simulink model "CA_CSE1_V1e_wo_LOSV2b"  (Simulink 7.3)
settings: Solver=ode3  StartTime=0.0  StopTime=Inf  FixedStep=0.1  RelTol=1e-3
undefined symbols (not defined in the file): eta1_0_real, v1_0_real, velocitySatValues1
libraries: simulink_extras x7, marine_gnc x5, simulink x5, dspinverses x2
(part 1 of 2)
settings Model: Creator=Dinh  LastModifiedBy=mcl  BufferReuse=off
settings DataIOCC: LimitDataPoints=off  SaveOutput=off  SaveTime=off
settings OptimizationCC: BlockReduction=off  BooleanDataType=off  ConditionallyExecuteInputs=off  OptimizeBlockIOStorage=off  BufferReuse=off  ExpressionFolding=off  LocalBlockOutputs=off  SimCompilerOptimization=On
settings SFSimCC: SimBuildMode=sf_nonincremental_build
settings RTWCC: SystemTargetFile=nidll.tlc  TemplateMakefile=nidll_vc.tmf  Description=NI Real-Time Target for Release 2007b or later  ProcessScript=nidll_make_rtw_hook
settings STFCustomTargetCC: MatFileLogging=on  SystemTargetFile=nidll.tlc

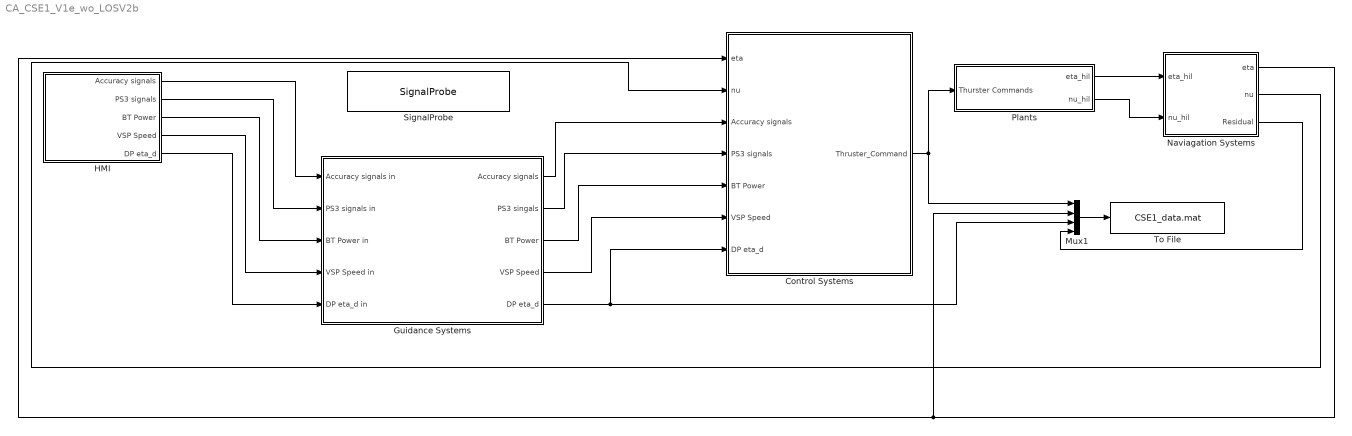
== system CA_CSE1_V1e_wo_LOSV2b ==
  Control Systems : Subsystem
  Guidance Systems : Subsystem
  HMI : Subsystem
  Mux1 : Mux
  Naviagation Systems : Subsystem
      settings: MinAlgLoopOccurrences=on
  Plants : Subsystem
  SignalProbe : S-Function  Description=Use this block with SIT.  FunctionName=SignalProbe  Parameters=1  EnableBusSupport=off
      settings: PreSaveFcn=NISIT_ModelVars;
      mask Description: The LabVIEW Simulation Interface Toolkit uses the SignalProbe block to probe the signals in the model. The SignalProbe block must be on the top level of the model hierarchy. You can have only one SignalProbe block per model file. Do not rename the SignalProbe block. Do not change the name of another model block to SignalProbe.
  To File : ToFile  Filename=CSE1_data.mat  MatrixName=cse1_data
  wires:
  Control Systems/1(Thruster_Command) -> Plants/1(Thurster Commands), Mux1/1
  HMI/2(PS3 signals) -> Guidance Systems/2(PS3 signals in)
  HMI/3(BT Power) -> Guidance Systems/3(BT Power in)
  HMI/4(VSP Speed) -> Guidance Systems/4(VSP Speed in)
  HMI/5(DP eta_d) -> Guidance Systems/5(DP eta_d in)
  Guidance Systems/2(PS3 singals) -> Control Systems/4(PS3 signals)
  Guidance Systems/3(BT Power) -> Control Systems/5(BT Power)
  Guidance Systems/4(VSP Speed) -> Control Systems/6(VSP Speed)
  Guidance Systems/5(DP eta_d) -> Control Systems/7(DP eta_d), Mux1/3
  Plants/1(eta_hil) -> Naviagation Systems/1(eta_hil)
  Plants/2(nu_hil) -> Naviagation Systems/2(nu_hil)
  Naviagation Systems/1(eta) -> Control Systems/1(eta), Mux1/2
  Naviagation Systems/2(nu) -> Control Systems/2(nu)
  Mux1/1 -> To File/1
  Guidance Systems/1(Accuracy signals) -> Control Systems/3(Accuracy signals)
  HMI/1(Accuracy signals) -> Guidance Systems/1(Accuracy signals in)
  Naviagation Systems/3(Residual) -> Mux1/4

== system CA_CSE1_V1e_wo_LOSV2b/Control Systems ==
  eta : Inport
  nu : Inport  Port=2
  Accuracy signals : Inport  Port=3
  PS3 signals : Inport  Port=4
  BT Power : Inport  Port=5
  VSP Speed : Inport  Port=6
  DP eta_d : Inport  Port=7
  Accuracy Control : Subsystem
  Control Switch : MultiPortSwitch  Inputs=4  zeroidx=on
  Control Mode : Constant  Value=0
  DP control : Subsystem
  Joystick Control : Subsystem
      settings: MinAlgLoopOccurrences=on
  Manual Thrust control : Subsystem
      settings: MinAlgLoopOccurrences=on
  Saturation : Saturate  UpperLimit=1.0  LowerLimit=-1.0
  if DP Control Mode : simulink/Logic and Bit Operations/Compare To Constant  SystemSampleTime=-1  relop===  const=3  LogicOutDataTypeMode=uint8
  Thruster_Command : Outport
  wires:
  PS3 signals/1 -> Manual Thrust control/1(PS3 Signals), Joystick Control/1(PS3 Signals)
  DP eta_d/1 -> DP control/1(eta_d)
  nu/1 -> DP control/3(nu)
  eta/1 -> DP control/2(eta)
  Control Mode/1 -> Control Switch/1, if DP Control Mode/1
  Control Switch/1 -> Saturation/1
  BT Power/1 -> Manual Thrust control/2(BT Power), Joystick Control/2(BT Power)
  VSP Speed/1 -> Manual Thrust control/3(VSP Speed), Joystick Control/3(VSP Speed)
  if DP Control Mode/1 -> DP control/Enable
  DP control/1(Thruster_Command_DP) -> Control Switch/5
  Joystick Control/1(Thruster_Command_Joystick) -> Control Switch/4
  Manual Thrust control/1(Thruster_Command_Manual) -> Control Switch/3
  Saturation/1 -> Thruster_Command/1
  Accuracy Control/1(Thruster Command Accuracy) -> Control Switch/2
  Accuracy signals/1 -> Accuracy Control/1(Accuracy signals)

== system CA_CSE1_V1e_wo_LOSV2b/Guidance Systems ==
  Accuracy signals in : Inport
  PS3 signals in : Inport  Port=2
  BT Power in : Inport  Port=3
  VSP Speed in : Inport  Port=4
  DP eta_d in : Inport  Port=5
  DP : Subsystem
  Demux1 : Demux  Outputs=3
  Mux : Mux  Inputs=3
  Terminator : Terminator
  psi_d : Gain  ParameterDataType=fixdt(1, 16)  ParameterScaling=2^0  OutDataType=fixdt(1, 16)  OutScaling=2^0
  x_d : Gain  ParameterDataType=fixdt(1, 16)  ParameterScaling=2^0  OutDataType=fixdt(1, 16)  OutScaling=2^0
  y_d : Gain  ParameterDataType=fixdt(1, 16)  ParameterScaling=2^0  OutDataType=fixdt(1, 16)  OutScaling=2^0
  Accuracy signals : Outport
  PS3 singals : Outport  Port=2
  BT Power : Outport  Port=3
  VSP Speed : Outport  Port=4
  DP eta_d : Outport  Port=5
  wires:
  DP eta_d in/1 -> DP/1(DP eta_d in)
  PS3 signals in/1 -> PS3 singals/1
  VSP Speed in/1 -> VSP Speed/1
  BT Power in/1 -> BT Power/1
  DP/1(DP eta_d) -> DP eta_d/1, Demux1/1
  Accuracy signals in/1 -> Accuracy signals/1
  x_d/1 -> Mux/1
  y_d/1 -> Mux/2
  psi_d/1 -> Mux/3
  Demux1/1 -> x_d/1
  Demux1/2 -> y_d/1
  Demux1/3 -> psi_d/1
  Mux/1 -> Terminator/1

== system CA_CSE1_V1e_wo_LOSV2b/HMI ==
  Accuracy control : Subsystem
  Battery Bow Thruster : Gain  ParameterDataType=fixdt(1, 16)  ParameterScaling=2^0  OutDataType=fixdt(1, 16)  OutScaling=2^0
  Battery Main : Gain  ParameterDataType=fixdt(1, 16)  ParameterScaling=2^0  OutDataType=fixdt(1, 16)  OutScaling=2^0
  Battery Servo : Gain  ParameterDataType=fixdt(1, 16)  ParameterScaling=2^0  OutDataType=fixdt(1, 16)  OutScaling=2^0
  DP input : Subsystem
  PS3 input : Subsystem
  SIT zAI0 : S-Function  Priority=1  FunctionName=NI_SIT_IO  Parameters=width dtype portnum stime stype btype  EnableBusSupport=off  mask(SIT Inport){portnum=1, width=-1, stime=-1, dtype=auto, stype=auto, btype=1}
      mask prompts: portnum "Port number:"; width "Port dimensions (-1 for dynamically sized):"; stime "Sample time (-1 for inherited):"; dtype "Data type:"; stype "Signal type:"; btype "Block type:"
      mask help: Use this inport on any level of nested subsystems to allow the LabVIEW Simulation Interface Toolkit to map hardware to it.
      mask init:
      | NI_SIT_IO_init;
      settings: CopyFcn=NI_SIT_IO_callbacks(1);  DeleteFcn=NI_SIT_IO_callbacks(2);
      mask StyleString: edit,edit,edit,popup(auto|double|single|int8|uint8|int16|uint16|int32|uint32|boolean),popup(auto|real|complex),edit
      mask CallbackString: NI_SIT_IO_callbacks(3);|||NI_SIT_IO_callbacks(4);||
      mask TabNameString: Parameters,Parameters,Parameters,Parameters,Parameters,Parameters
      mask Display:
      | patch([-x x], [-y y], [.90980 .81960 .32156]);
      | plot([0 -x x 0], [rad -y y rad]);
      | fprintf('SIT%d', portnum);
  SIT zAI1 : S-Function  Priority=2  FunctionName=NI_SIT_IO  Parameters=width dtype portnum stime stype btype  EnableBusSupport=off  mask(SIT Inport){portnum=2, width=-1, stime=-1, dtype=auto, stype=auto, btype=1}
      mask prompts: portnum "Port number:"; width "Port dimensions (-1 for dynamically sized):"; stime "Sample time (-1 for inherited):"; dtype "Data type:"; stype "Signal type:"; btype "Block type:"
      mask help: Use this inport on any level of nested subsystems to allow the LabVIEW Simulation Interface Toolkit to map hardware to it.
      mask init:
      | NI_SIT_IO_init;
      settings: CopyFcn=NI_SIT_IO_callbacks(1);  DeleteFcn=NI_SIT_IO_callbacks(2);
      mask StyleString: edit,edit,edit,popup(auto|double|single|int8|uint8|int16|uint16|int32|uint32|boolean),popup(auto|real|complex),edit
      mask CallbackString: NI_SIT_IO_callbacks(3);|||NI_SIT_IO_callbacks(4);||
      mask TabNameString: Parameters,Parameters,Parameters,Parameters,Parameters,Parameters
      mask Display:
      | patch([-x x], [-y y], [.90980 .81960 .32156]);
      | plot([0 -x x 0], [rad -y y rad]);
      | fprintf('SIT%d', portnum);
  SIT zAI2 : S-Function  Priority=3  FunctionName=NI_SIT_IO  Parameters=width dtype portnum stime stype btype  EnableBusSupport=off  mask(SIT Inport){portnum=3, width=-1, stime=-1, dtype=auto, stype=auto, btype=1}
      mask prompts: portnum "Port number:"; width "Port dimensions (-1 for dynamically sized):"; stime "Sample time (-1 for inherited):"; dtype "Data type:"; stype "Signal type:"; btype "Block type:"
      mask help: Use this inport on any level of nested subsystems to allow the LabVIEW Simulation Interface Toolkit to map hardware to it.
      mask init:
      | NI_SIT_IO_init;
      settings: CopyFcn=NI_SIT_IO_callbacks(1);  DeleteFcn=NI_SIT_IO_callbacks(2);
      mask StyleString: edit,edit,edit,popup(auto|double|single|int8|uint8|int16|uint16|int32|uint32|boolean),popup(auto|real|complex),edit
      mask CallbackString: NI_SIT_IO_callbacks(3);|||NI_SIT_IO_callbacks(4);||
      mask TabNameString: Parameters,Parameters,Parameters,Parameters,Parameters,Parameters
      mask Display:
      | patch([-x x], [-y y], [.90980 .81960 .32156]);
      | plot([0 -x x 0], [rad -y y rad]);
      | fprintf('SIT%d', portnum);
  Terminator Bow Thruster Battery : Terminator
  Terminator Main Battery : Terminator
  Terminator Servo Battery : Terminator
  Accuracy signals : Outport
  PS3 signals : Outport  Port=2
  BT Power : Outport  Port=3
  VSP Speed : Outport  Port=4
  DP eta_d : Outport  Port=5
  wires:
  PS3 input/1(PS3) -> PS3 signals/1
  DP input/1(DP eta_d) -> DP eta_d/1
  PS3 input/3(VSP Speed) -> VSP Speed/1
  PS3 input/2(BP power) -> BT Power/1
  SIT zAI0/1 -> Battery Bow Thruster/1
  SIT zAI1/1 -> Battery Servo/1
  SIT zAI2/1 -> Battery Main/1
  Battery Bow Thruster/1 -> Terminator Bow Thruster Battery/1
  Battery Servo/1 -> Terminator Servo Battery/1
  Battery Main/1 -> Terminator Main Battery/1
  Accuracy control/1(Accuracy signals) -> Accuracy signals/1

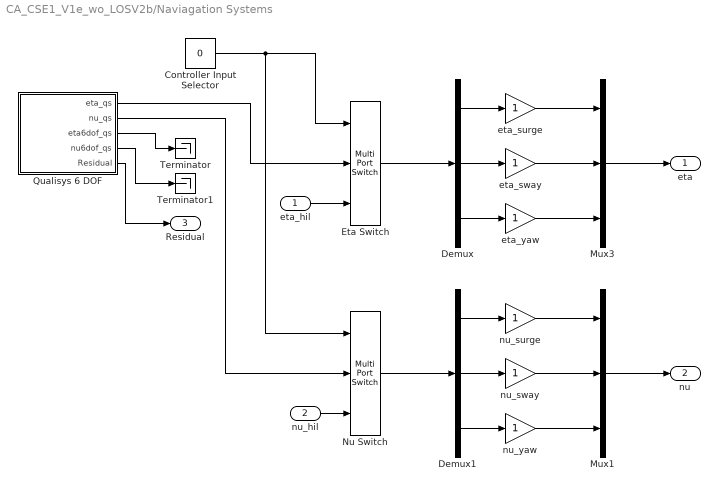
== system CA_CSE1_V1e_wo_LOSV2b/Naviagation Systems ==
  eta_hil : Inport
  nu_hil : Inport  Port=2
  Controller Input Selector : Constant  Value=0
  Demux : Demux  Outputs=3
  Demux1 : Demux  Outputs=3
  Eta Switch : MultiPortSwitch  Inputs=2  zeroidx=on
  Mux1 : Mux  Inputs=3
  Mux3 : Mux  Inputs=3
  Nu Switch : MultiPortSwitch  Inputs=2  zeroidx=on
  Qualisys 6 DOF : Subsystem
  Terminator : Terminator
  Terminator1 : Terminator
  eta_surge : Gain  ParameterDataType=fixdt(1, 16)  ParameterScaling=2^0  OutDataType=fixdt(1, 16)  OutScaling=2^0
  eta_sway : Gain  ParameterDataType=fixdt(1, 16)  ParameterScaling=2^0  OutDataType=fixdt(1, 16)  OutScaling=2^0
  eta_yaw : Gain  ParameterDataType=fixdt(1, 16)  ParameterScaling=2^0  OutDataType=fixdt(1, 16)  OutScaling=2^0
  nu_surge : Gain  ParameterDataType=fixdt(1, 16)  ParameterScaling=2^0  OutDataType=fixdt(1, 16)  OutScaling=2^0
  nu_sway : Gain  ParameterDataType=fixdt(1, 16)  ParameterScaling=2^0  OutDataType=fixdt(1, 16)  OutScaling=2^0
  nu_yaw : Gain  ParameterDataType=fixdt(1, 16)  ParameterScaling=2^0  OutDataType=fixdt(1, 16)  OutScaling=2^0
  eta : Outport
  nu : Outport  Port=2
  Residual : Outport  Port=3
  wires:
  Controller Input Selector/1 -> Eta Switch/1, Nu Switch/1
  Qualisys 6 DOF/1(eta_qs) -> Eta Switch/2
  Qualisys 6 DOF/2(nu_qs) -> Nu Switch/2
  eta_hil/1 -> Eta Switch/3
  nu_hil/1 -> Nu Switch/3
  Qualisys 6 DOF/3(eta6dof_qs) -> Terminator/1
  Qualisys 6 DOF/4(nu6dof_qs) -> Terminator1/1
  Demux/1 -> eta_surge/1
  Demux/2 -> eta_sway/1
  Demux/3 -> eta_yaw/1
  eta_surge/1 -> Mux3/1
  eta_yaw/1 -> Mux3/3
  eta_sway/1 -> Mux3/2
  Mux3/1 -> eta/1
  Demux1/1 -> nu_surge/1
  Demux1/2 -> nu_sway/1
  Demux1/3 -> nu_yaw/1
  nu_surge/1 -> Mux1/1
  nu_sway/1 -> Mux1/2
  nu_yaw/1 -> Mux1/3
  Mux1/1 -> nu/1
  Nu Switch/1 -> Demux1/1
  Eta Switch/1 -> Demux/1
  Qualisys 6 DOF/5(Residual) -> Residual/1

== system CA_CSE1_V1e_wo_LOSV2b/Plants ==
  Thurster Commands : Inport
  BT power limit plant : Gain  ParameterDataType=fixdt(1, 16)  ParameterScaling=2^0  OutDataType=fixdt(1, 16)  OutScaling=2^0
  CSE1 : Subsystem
  Demux : Demux  Outputs=7
  Enable CSE1 : Constant  Value=0
  Enable Linear Simulator : Constant  Value=0
  Linear Simulator : Subsystem
      settings: MinAlgLoopOccurrences=on
  Mux : Mux  Inputs=7
  VSP speed plant : Gain  ParameterDataType=fixdt(1, 16)  ParameterScaling=2^0  OutDataType=fixdt(1, 16)  OutScaling=2^0
  u_1 plant : Gain  ParameterDataType=fixdt(1, 16)  ParameterScaling=2^0  OutDataType=fixdt(1, 16)  OutScaling=2^0
  u_2 plant : Gain  ParameterDataType=fixdt(1, 16)  ParameterScaling=2^0  OutDataType=fixdt(1, 16)  OutScaling=2^0
  u_3 plant : Gain  ParameterDataType=fixdt(1, 16)  ParameterScaling=2^0  OutDataType=fixdt(1, 16)  OutScaling=2^0
  u_4 plant : Gain  ParameterDataType=fixdt(1, 16)  ParameterScaling=2^0  OutDataType=fixdt(1, 16)  OutScaling=2^0
  u_5 plant : Gain  ParameterDataType=fixdt(1, 16)  ParameterScaling=2^0  OutDataType=fixdt(1, 16)  OutScaling=2^0
  eta_hil : Outport
  nu_hil : Outport  Port=2
  wires:
  Linear Simulator/1(eta_hil) -> eta_hil/1
  Linear Simulator/2(nu_hil) -> nu_hil/1
  Enable CSE1/1 -> CSE1/Enable
  Enable Linear Simulator/1 -> Linear Simulator/Enable
  Thurster Commands/1 -> Demux/1
  Mux/1 -> CSE1/1(Thruster_Commands), Linear Simulator/1(Thruster commands)
  Demux/1 -> u_1 plant/1
  Demux/2 -> u_2 plant/1
  Demux/3 -> u_3 plant/1
  Demux/4 -> u_4 plant/1
  u_4 plant/1 -> Mux/4
  u_1 plant/1 -> Mux/1
  u_2 plant/1 -> Mux/2
  u_3 plant/1 -> Mux/3
  Demux/5 -> u_5 plant/1
  Demux/6 -> BT power limit plant/1
  Demux/7 -> VSP speed plant/1
  u_5 plant/1 -> Mux/5
  BT power limit plant/1 -> Mux/6
  VSP speed plant/1 -> Mux/7

== system CA_CSE1_V1e_wo_LOSV2b/Control Systems/Accuracy Control ==
  Accuracy signals : Inport
  Thruster Command Accuracy : Outport
  wires:
  Accuracy signals/1 -> Thruster Command Accuracy/1

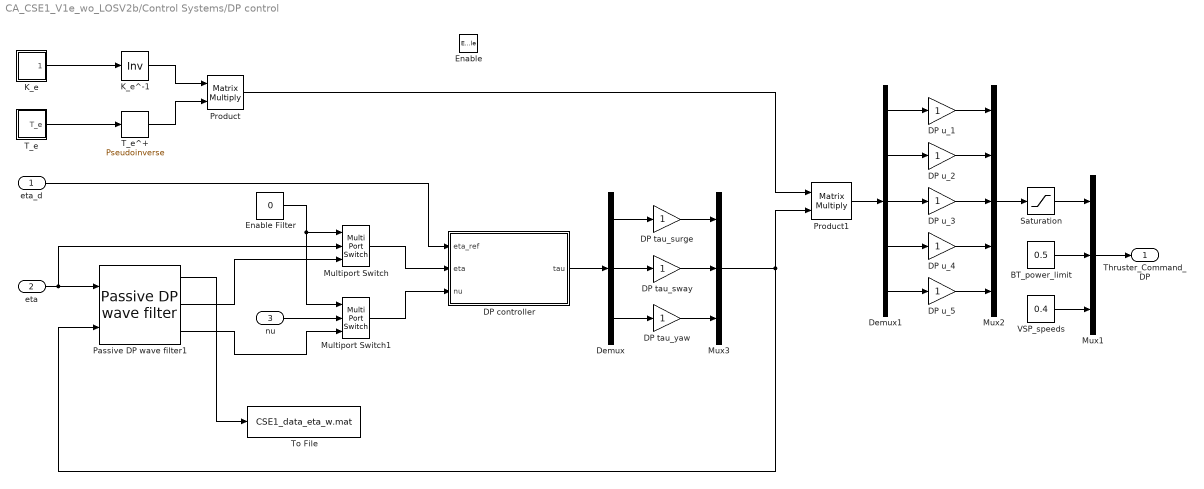
== system CA_CSE1_V1e_wo_LOSV2b/Control Systems/DP control ==
  eta_d : Inport
  eta : Inport  Port=2
  nu : Inport  Port=3
  Enable : EnablePort  StatesWhenEnabling=reset
  BT_power_limit : Constant  Value=0.5
  DP controller : Subsystem  mask(Nonlinear DP Controller){Kp=(0.1)^2*[25.8000 0  0;  0  33.8000  1.0115;  0  1.0115  2.7600 ], Kd=2*0.8*0.1*[25.8000 0  0;  0  33.8000  1.0115;  0  1.0115  2.7600 ], Ki=(0.1^3/10)*[25.8000 0  0;  0  33.8000  1.0115;  0  1.0115  2.7600 ]}
      mask prompts: Kp "Proportional Gain Matrix: Kp"; Kd "Derivative Gain Matrix: Kd"; Ki "Integral Gain Matrix: Ki"
      mask help: Nonlinear PID controller for Set-Point Reulation in Surge, Sway and Yaw
      mask Help:
      | The nonlinear  PID controller uses the rotation matrix in yaw for proper scaling of the surge, sway and yaw gains as a function of the yaw angle.
      | INPUTS: (1) eta_ref, (2) eta, (3) nu. OUPUTS: (1) tau.
      mask Display: disp('Nonlinear PID\n set-point controller')
  DP tau_surge : Gain  ParameterDataType=fixdt(1, 16)  ParameterScaling=2^0  OutDataType=fixdt(1, 16)  OutScaling=2^0
  DP tau_sway : Gain  ParameterDataType=fixdt(1, 16)  ParameterScaling=2^0  OutDataType=fixdt(1, 16)  OutScaling=2^0
  DP tau_yaw : Gain  ParameterDataType=fixdt(1, 16)  ParameterScaling=2^0  OutDataType=fixdt(1, 16)  OutScaling=2^0
  DP u_{1..5} (5 alike) : Gain  ParameterDataType=fixdt(1, 16)  ParameterScaling=2^0  OutDataType=fixdt(1, 16)  OutScaling=2^0
  Demux : Demux  Outputs=3
  Demux1 : Demux  Outputs=5
  Enable Filter : Constant  Value=0
  K_e : Subsystem
  K_e^-1 : Product  Inputs=/  Multiplication=Matrix(*)
  Multiport Switch : MultiPortSwitch  Inputs=2  zeroidx=on
  Multiport Switch1 : MultiPortSwitch  Inputs=2  zeroidx=on
  Mux1 : Mux  Inputs=3
  Mux2 : Mux  Inputs=5
  Mux3 : Mux  Inputs=3
  Passive DP wave filter1 : marine_gnc/Navigation/Observers/Passive DP wave filter  SystemSampleTime=-1  lambda=0.1*diag([1 1 1])  w_o=diag([0.8 0.8 0.8])  K4=0.1*diag([1 1 0.1])  K3=0.1*diag([1 1 0.1])  w_c=1.3*diag([0.8 0.8 0.8])  T_b=diag([100 100 100])  M="[ 25.8000   0    0;   0   33.8000   1.0115; 0   1.0115    2.7600 ]"  D="[2 0  0;  0 7 0.1; 0 0.1 0.5]"
  Product : Product  Multiplication=Matrix(*)  RndMeth=Zero
  Product1 : Product  Multiplication=Matrix(*)  RndMeth=Zero
  Saturation : Saturate  UpperLimit=1.0  LowerLimit=-1.0
  T_e : Subsystem
  T_e^+ : dspinverses/Pseudoinverse  wanterr=off
  To File : ToFile  Filename=CSE1_data_eta_w.mat  MatrixName=cse1_data
  VSP_speeds : Constant  Value=0.4
  Thruster_Command_DP : Outport  InitialOutput=[0;0;0;0;0;0;0]
  wires:
  Product/1 -> Product1/1
  Mux1/1 -> Thruster_Command_DP/1
  eta_d/1 -> DP controller/1(eta_ref)
  eta/1 -> Passive DP wave filter1/1, Multiport Switch/2
  nu/1 -> Multiport Switch1/2
  Multiport Switch/1 -> DP controller/2(eta)
  Multiport Switch1/1 -> DP controller/3(nu)
  Passive DP wave filter1/2 -> Multiport Switch/3
  Passive DP wave filter1/3 -> Multiport Switch1/3
  Enable Filter/1 -> Multiport Switch/1, Multiport Switch1/1
  Saturation/1 -> Mux1/1
  Passive DP wave filter1/1 -> To File/1
  T_e/1(T_e) -> T_e^+/1
  K_e/1(K_e) -> K_e^-1/1
  K_e^-1/1 -> Product/1
  T_e^+/1 -> Product/2
  BT_power_limit/1 -> Mux1/2
  VSP_speeds/1 -> Mux1/3
  Demux/1 -> DP tau_surge/1
  Demux/2 -> DP tau_sway/1
  Demux/3 -> DP tau_yaw/1
  DP tau_surge/1 -> Mux3/1
  DP tau_yaw/1 -> Mux3/3
  DP tau_sway/1 -> Mux3/2
  DP controller/1(tau) -> Demux/1
  Mux3/1 -> Product1/2, Passive DP wave filter1/2
  Demux1/1 -> DP u_1/1
  Demux1/2 -> DP u_2/1
  Demux1/3 -> DP u_3/1
  DP u_1/1 -> Mux2/1
  DP u_3/1 -> Mux2/3
  DP u_2/1 -> Mux2/2
  Demux1/4 -> DP u_4/1
  Demux1/5 -> DP u_5/1
  DP u_4/1 -> Mux2/4
  DP u_5/1 -> Mux2/5
  Product1/1 -> Demux1/1
  Mux2/1 -> Saturation/1

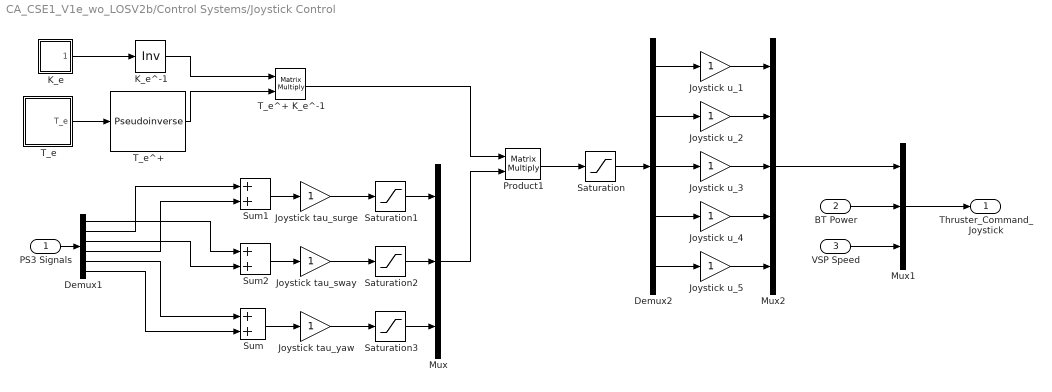
== system CA_CSE1_V1e_wo_LOSV2b/Control Systems/Joystick Control ==
  PS3 Signals : Inport
  BT Power : Inport  Port=2
  VSP Speed : Inport  Port=3
  Demux1 : Demux  Outputs=6
  Demux2 : Demux  Outputs=5
  Joystick tau_surge : Gain
  Joystick tau_sway : Gain
  Joystick tau_yaw : Gain
  Joystick u_{1..5} (5 alike) : Gain  ParameterDataType=fixdt(1, 16)  ParameterScaling=2^0  OutDataType=fixdt(1, 16)  OutScaling=2^0
  K_e : Subsystem
  K_e^-1 : Product  Inputs=/  Multiplication=Matrix(*)
  Mux : Mux  Inputs=3
  Mux1 : Mux  Inputs=3
  Mux2 : Mux  Inputs=5
  Product1 : Product  Multiplication=Matrix(*)  RndMeth=Zero
  Saturation{,1..3} (4 alike) : Saturate  UpperLimit=1.0  LowerLimit=-1.0
  Sum : Sum
  Sum1 : Sum
  Sum2 : Sum
  T_e : Subsystem
  T_e^+ : dspinverses/Pseudoinverse  wanterr=off
  T_e^+ K_e^-1 : Product  Multiplication=Matrix(*)  RndMeth=Zero
  Thruster_Command_Joystick : Outport
  wires:
  PS3 Signals/1 -> Demux1/1
  Demux1/5 -> Sum/1
  Demux1/6 -> Sum/2
  Sum/1 -> Joystick tau_yaw/1
  T_e^+ K_e^-1/1 -> Product1/1
  Mux/1 -> Product1/2
  Mux1/1 -> Thruster_Command_Joystick/1
  BT Power/1 -> Mux1/2
  VSP Speed/1 -> Mux1/3
  Product1/1 -> Saturation/1
  T_e/1(T_e) -> T_e^+/1
  K_e/1(K_e) -> K_e^-1/1
  K_e^-1/1 -> T_e^+ K_e^-1/1
  T_e^+/1 -> T_e^+ K_e^-1/2
  Demux1/4 -> Sum1/2
  Demux1/2 -> Sum1/1
  Sum1/1 -> Joystick tau_surge/1
  Demux1/1 -> Sum2/1
  Demux1/3 -> Sum2/2
  Sum2/1 -> Joystick tau_sway/1
  Demux2/1 -> Joystick u_1/1
  Demux2/2 -> Joystick u_2/1
  Demux2/3 -> Joystick u_3/1
  Joystick u_1/1 -> Mux2/1
  Joystick u_3/1 -> Mux2/3
  Joystick u_2/1 -> Mux2/2
  Demux2/4 -> Joystick u_4/1
  Demux2/5 -> Joystick u_5/1
  Joystick u_4/1 -> Mux2/4
  Joystick u_5/1 -> Mux2/5
  Saturation/1 -> Demux2/1
  Mux2/1 -> Mux1/1
  Joystick tau_surge/1 -> Saturation1/1
  Saturation1/1 -> Mux/1
  Joystick tau_sway/1 -> Saturation2/1
  Saturation2/1 -> Mux/2
  Joystick tau_yaw/1 -> Saturation3/1
  Saturation3/1 -> Mux/3

== system CA_CSE1_V1e_wo_LOSV2b/Control Systems/Manual Thrust control ==
  PS3 Signals : Inport
  BT Power : Inport  Port=2
  VSP Speed : Inport  Port=3
  Add : Sum  Inputs=|++
  Demux : Demux  Outputs=6
  Mux : Mux  Inputs=7
  PS3 u_{1..5} (5 alike) : Gain  ParameterDataType=fixdt(1, 16)  ParameterScaling=2^0  OutDataType=fixdt(1, 16)  OutScaling=2^0
  Thruster_Command_Manual : Outport
  wires:
  PS3 Signals/1 -> Demux/1
  Demux/1 -> PS3 u_2/1  "Left/Right position of Left Joystick"
  Demux/2 -> PS3 u_1/1  "Up/Down position of Left Joystick"
  Demux/3 -> PS3 u_4/1  "Left/Right position of Right Joystick"
  Demux/4 -> PS3 u_3/1  "Up/Down position of Right Joystick"
  Demux/5 -> Add/1  "L2 signal"
  Demux/6 -> Add/2  "R2 signal"
  VSP Speed/1 -> Mux/7  "VPS Speed"
  BT Power/1 -> Mux/6  "Bow Thruster Limit"
  Add/1 -> PS3 u_5/1  "Bow Thruster direction"
  Mux/1 -> Thruster_Command_Manual/1
  PS3 u_1/1 -> Mux/1
  PS3 u_2/1 -> Mux/2
  PS3 u_5/1 -> Mux/5
  PS3 u_4/1 -> Mux/4
  PS3 u_3/1 -> Mux/3

== system CA_CSE1_V1e_wo_LOSV2b/Guidance Systems/DP ==
  DP eta_d in : Inport
  Demux : Demux  Outputs=3
  Demux1 : Demux  Outputs=3
  Enable eta_d LPF : Constant  Value=0  OutDataType=fixdt(1, 16)  OutScaling=2^0
  Multiport Switch : MultiPortSwitch  Inputs=2  zeroidx=on  OutDataType=fixdt(1, 16)  OutScaling=2^0
  Mux : Mux  Inputs=3
  Mux1 : Mux  Inputs=3
  Terminator : Terminator
  Transfer Fcn : TransferFcn  Numerator=[0.1]  Denominator=[1 0.1]
  Transfer Fcn1 : TransferFcn  Numerator=[0.1]  Denominator=[1 0.1]
  Transfer Fcn2 : TransferFcn  Numerator=[0.1]  Denominator=[1 0.1]
  eta_d DP E : Gain  ParameterDataType=fixdt(1, 16)  ParameterScaling=2^0  OutDataType=fixdt(1, 16)  OutScaling=2^0
  eta_d DP N : Gain  ParameterDataType=fixdt(1, 16)  ParameterScaling=2^0  OutDataType=fixdt(1, 16)  OutScaling=2^0
  eta_d DP Psi : Gain  ParameterDataType=fixdt(1, 16)  ParameterScaling=2^0  OutDataType=fixdt(1, 16)  OutScaling=2^0
  eta_d Psi deg : Gain  Gain=180/pi  ParameterDataType=fixdt(1, 16)  ParameterScaling=2^0  OutDataType=fixdt(1, 16)  OutScaling=2^0
  DP eta_d : Outport
  wires:
  Enable eta_d LPF/1 -> Multiport Switch/1
  Mux1/1 -> Multiport Switch/3
  Demux/1 -> Transfer Fcn/1
  Transfer Fcn/1 -> Mux1/1
  Demux/2 -> Transfer Fcn1/1
  Transfer Fcn1/1 -> Mux1/2
  Demux/3 -> Transfer Fcn2/1
  Transfer Fcn2/1 -> Mux1/3
  DP eta_d in/1 -> Multiport Switch/2, Demux/1
  Multiport Switch/1 -> Demux1/1
  eta_d DP N/1 -> Mux/1
  eta_d DP E/1 -> Mux/2
  eta_d DP Psi/1 -> Mux/3
  Demux1/1 -> eta_d DP N/1
  Demux1/2 -> eta_d DP E/1
  Demux1/3 -> eta_d DP Psi/1, eta_d Psi deg/1
  Mux/1 -> DP eta_d/1
  eta_d Psi deg/1 -> Terminator/1

== system CA_CSE1_V1e_wo_LOSV2b/HMI/Accuracy control ==
  Accuracy  BT power : Constant  Value=0
  Accuracy  VSP speed : Constant  Value=0
  Accuracy u_{1..5} (5 alike) : Gain  ParameterDataType=fixdt(1, 16)  ParameterScaling=2^0  OutDataType=fixdt(1, 16)  OutScaling=2^0
  Mux2 : Mux  Inputs=7
  u{1..5} (5 alike) : Constant  Value=0
  Accuracy signals : Outport
  wires:
  u1/1 -> Accuracy u_1/1
  u2/1 -> Accuracy u_2/1
  u3/1 -> Accuracy u_3/1
  Accuracy u_1/1 -> Mux2/1
  Accuracy u_3/1 -> Mux2/3
  Accuracy u_2/1 -> Mux2/2
  u4/1 -> Accuracy u_4/1
  u5/1 -> Accuracy u_5/1
  Accuracy u_4/1 -> Mux2/4
  Accuracy u_5/1 -> Mux2/5
  Mux2/1 -> Accuracy signals/1
  Accuracy  BT power/1 -> Mux2/6
  Accuracy  VSP speed/1 -> Mux2/7

== system CA_CSE1_V1e_wo_LOSV2b/HMI/DP input ==
  Degrees to Radians : simulink_extras/Transformations/Degrees to Radians  SystemSampleTime=-1
  Mux : Mux  Inputs=3
  psi_d : Constant  Value=0
  x_d : Constant  Value=0
  y_d : Constant  Value=0
  DP eta_d : Outport
  wires:
  x_d/1 -> Mux/1
  y_d/1 -> Mux/2
  Mux/1 -> DP eta_d/1
  psi_d/1 -> Degrees to Radians/1
  Degrees to Radians/1 -> Mux/3

== system CA_CSE1_V1e_wo_LOSV2b/HMI/PS3 input ==
  note: Direct signals from PS3 controller
  PS3 signals : Subsystem
  PS3_BT_Power : Constant  Value=0
  PS3_VSP_Speed : Constant  Value=0
  PS3 : Outport
  BP power : Outport  Port=2
  VSP Speed : Outport  Port=3
  wires:
  PS3_VSP_Speed/1 -> VSP Speed/1  "Voith Schnider Propeller Speed"
  PS3_BT_Power/1 -> BP power/1  "Bow Thruster Power limit"
  PS3 signals/1(PS3 signals) -> PS3/1

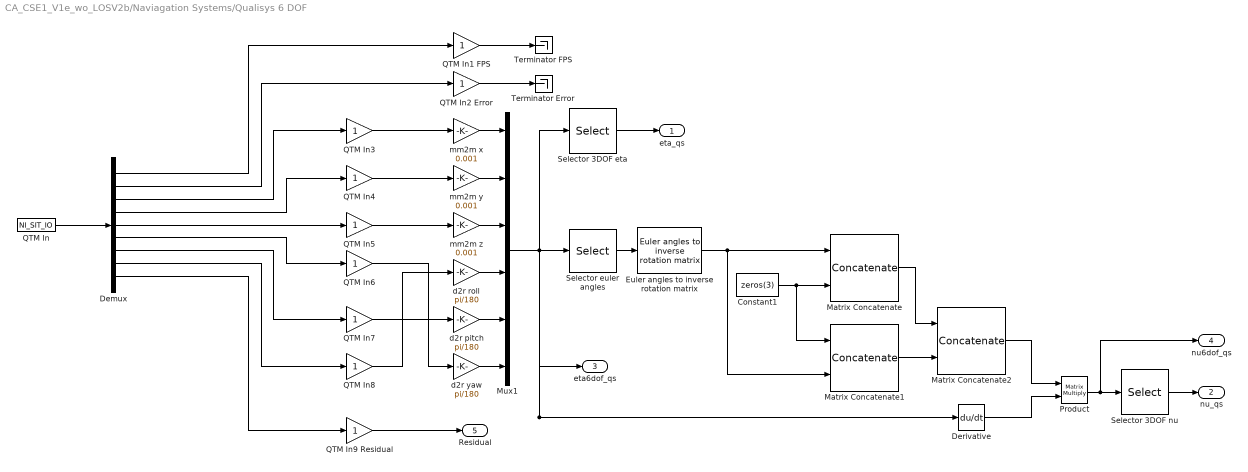
== system CA_CSE1_V1e_wo_LOSV2b/Naviagation Systems/Qualisys 6 DOF ==
  Constant1 : Constant  Value=zeros(3)
  Demux : Demux  Outputs=9
  Derivative : Derivative
  Euler angles to inverse rotation matrix : marine_gnc/Models/ Kinematics/Euler angles to inverse rotation matrix  SystemSampleTime=-1
  Matrix Concatenate : Concatenate  Mode=Multidimensional array
  Matrix Concatenate1 : Concatenate  Mode=Multidimensional array
  Matrix Concatenate2 : Concatenate  Mode=Multidimensional array  ConcatenateDimension=2
  Mux1 : Mux  Inputs=6
  Product : Product  Multiplication=Matrix(*)  RndMeth=Zero
  QTM In : S-Function  Priority=1  FunctionName=NI_SIT_IO  Parameters=width dtype portnum stime stype btype  EnableBusSupport=off  mask(SIT Inport){portnum=1, width=9, stime=-1, dtype=auto, stype=auto, btype=1}
      mask prompts: portnum "Port number:"; width "Port dimensions (-1 for dynamically sized):"; stime "Sample time (-1 for inherited):"; dtype "Data type:"; stype "Signal type:"; btype "Block type:"
      mask help: Use this inport on any level of nested subsystems to allow the LabVIEW Simulation Interface Toolkit to map hardware to it.
      mask init:
      | NI_SIT_IO_init;
      settings: CopyFcn=NI_SIT_IO_callbacks(1);  DeleteFcn=NI_SIT_IO_callbacks(2);
      mask StyleString: edit,edit,edit,popup(auto|double|single|int8|uint8|int16|uint16|int32|uint32|boolean),popup(auto|real|complex),edit
      mask CallbackString: NI_SIT_IO_callbacks(3);|||NI_SIT_IO_callbacks(4);||
      mask TabNameString: Parameters,Parameters,Parameters,Parameters,Parameters,Parameters
      mask Display:
      | patch([-x x], [-y y], [.90980 .81960 .32156]);
      | plot([0 -x x 0], [rad -y y rad]);
      | fprintf('SIT%d', portnum);
  QTM In1 FPS : Gain  ParameterDataType=fixdt(1, 16)  ParameterScaling=2^0  OutDataType=fixdt(1, 16)  OutScaling=2^0
  QTM In2 Error : Gain  ParameterDataType=fixdt(1, 16)  ParameterScaling=2^0  OutDataType=fixdt(1, 16)  OutScaling=2^0
  QTM In{3..8} (6 alike) : Gain  ParameterDataType=fixdt(1, 16)  ParameterScaling=2^0  OutDataType=fixdt(1, 16)  OutScaling=2^0
  QTM In9 Residual : Gain  ParameterDataType=fixdt(1, 16)  ParameterScaling=2^0  OutDataType=fixdt(1, 16)  OutScaling=2^0
  Selector 3DOF eta : Selector  InputPortWidth=6  IndexOptions=Index vector (dialog)  Indices=[1 2 6]  OutputSizes=1
  Selector 3DOF nu : Selector  InputPortWidth=6  IndexOptions=Index vector (dialog)  Indices=[1 2 6]  OutputSizes=1
  Selector euler angles : Selector  InputPortWidth=6  IndexOptions=Index vector (dialog)  Indices=[4 5 6]  OutputSizes=1
  Terminator Error : Terminator
  Terminator FPS : Terminator
  d2r pitch : Gain  Gain=pi/180  ParameterDataType=fixdt(1, 16)  ParameterScaling=2^0  OutDataType=fixdt(1, 16)  OutScaling=2^0
  d2r roll : Gain  Gain=pi/180  ParameterDataType=fixdt(1, 16)  ParameterScaling=2^0  OutDataType=fixdt(1, 16)  OutScaling=2^0
  d2r yaw : Gain  Gain=pi/180  ParameterDataType=fixdt(1, 16)  ParameterScaling=2^0  OutDataType=fixdt(1, 16)  OutScaling=2^0
  mm2m x : Gain  Gain=0.001
  mm2m y : Gain  Gain=0.001
  mm2m z : Gain  Gain=0.001
  eta_qs : Outport
  nu_qs : Outport  Port=2
  eta6dof_qs : Outport  Port=3
  nu6dof_qs : Outport  Port=4
  Residual : Outport  Port=5
  wires:
  Mux1/1 -> Selector euler angles/1, Selector 3DOF eta/1, Derivative/1, eta6dof_qs/1
  Selector 3DOF eta/1 -> eta_qs/1
  Euler angles to inverse rotation matrix/1 -> Matrix Concatenate/1, Matrix Concatenate1/2
  Matrix Concatenate/1 -> Matrix Concatenate2/1
  Matrix Concatenate1/1 -> Matrix Concatenate2/2
  Matrix Concatenate2/1 -> Product/1
  Derivative/1 -> Product/2
  Constant1/1 -> Matrix Concatenate/2, Matrix Concatenate1/1
  mm2m z/1 -> Mux1/3
  mm2m y/1 -> Mux1/2
  mm2m x/1 -> Mux1/1
  d2r yaw/1 -> Mux1/6
  d2r pitch/1 -> Mux1/5
  d2r roll/1 -> Mux1/4
  Selector euler angles/1 -> Euler angles to inverse rotation matrix/1
  Product/1 -> Selector 3DOF nu/1, nu6dof_qs/1
  Selector 3DOF nu/1 -> nu_qs/1
  QTM In1 FPS/1 -> Terminator FPS/1
  QTM In2 Error/1 -> Terminator Error/1
  QTM In/1 -> Demux/1
  Demux/1 -> QTM In1 FPS/1
  Demux/2 -> QTM In2 Error/1
  Demux/3 -> QTM In3/1
  Demux/4 -> QTM In4/1
  Demux/5 -> QTM In5/1
  Demux/6 -> QTM In6/1
  Demux/7 -> QTM In7/1
  Demux/8 -> QTM In8/1
  Demux/9 -> QTM In9 Residual/1
  QTM In3/1 -> mm2m x/1
  QTM In4/1 -> mm2m y/1
  QTM In5/1 -> mm2m z/1
  QTM In7/1 -> d2r pitch/1
  QTM In6/1 -> d2r yaw/1
  QTM In8/1 -> d2r roll/1
  QTM In9 Residual/1 -> Residual/1

== system CA_CSE1_V1e_wo_LOSV2b/Plants/CSE1 ==
  Thruster_Commands : Inport
  Enable : EnablePort  StatesWhenEnabling=reset
  Bow Thruster : Subsystem
  CSE1 tau_surge : Gain  ParameterDataType=fixdt(1, 16)  ParameterScaling=2^0  OutDataType=fixdt(1, 16)  OutScaling=2^0
  CSE1 tau_sway : Gain  ParameterDataType=fixdt(1, 16)  ParameterScaling=2^0  OutDataType=fixdt(1, 16)  OutScaling=2^0
  CSE1 tau_yaw : Gain  ParameterDataType=fixdt(1, 16)  ParameterScaling=2^0  OutDataType=fixdt(1, 16)  OutScaling=2^0
  Demux : Demux  Outputs=7
  Demux1 : Demux  Outputs=3
  K_e : Subsystem
  Mux : Mux  Inputs=5
  T_e : Subsystem
  Terminator : Terminator
  Terminator1 : Terminator
  Terminator2 : Terminator
  "Voith Schneider Propeller " : Subsystem
  tau_cse1 : Product  Inputs=3  Multiplication=Matrix(*)  RndMeth=Zero
  wires:
  Thruster_Commands/1 -> Demux/1
  Demux/1 -> "Voith Schneider Propeller "/1(Port VSP y u_1), Mux/1
  Demux/2 -> "Voith Schneider Propeller "/2(Port VSP x u_2), Mux/2
  Demux/3 -> "Voith Schneider Propeller "/3(Starboard VSP y u_3), Mux/3
  Demux/4 -> "Voith Schneider Propeller "/4(Starboard VSP x u_4), Mux/4
  Demux/7 -> "Voith Schneider Propeller "/5(VSP Speed)
  Demux/5 -> Bow Thruster/1(Bow Thruster Direction u_5), Mux/5
  Demux/6 -> Bow Thruster/2(Bow Thruster Power)
  Demux1/1 -> CSE1 tau_surge/1
  Demux1/2 -> CSE1 tau_sway/1
  Demux1/3 -> CSE1 tau_yaw/1
  Mux/1 -> tau_cse1/3
  tau_cse1/1 -> Demux1/1
  T_e/1(T_e) -> tau_cse1/1
  K_e/1(K_e) -> tau_cse1/2
  CSE1 tau_surge/1 -> Terminator/1
  CSE1 tau_sway/1 -> Terminator1/1
  CSE1 tau_yaw/1 -> Terminator2/1

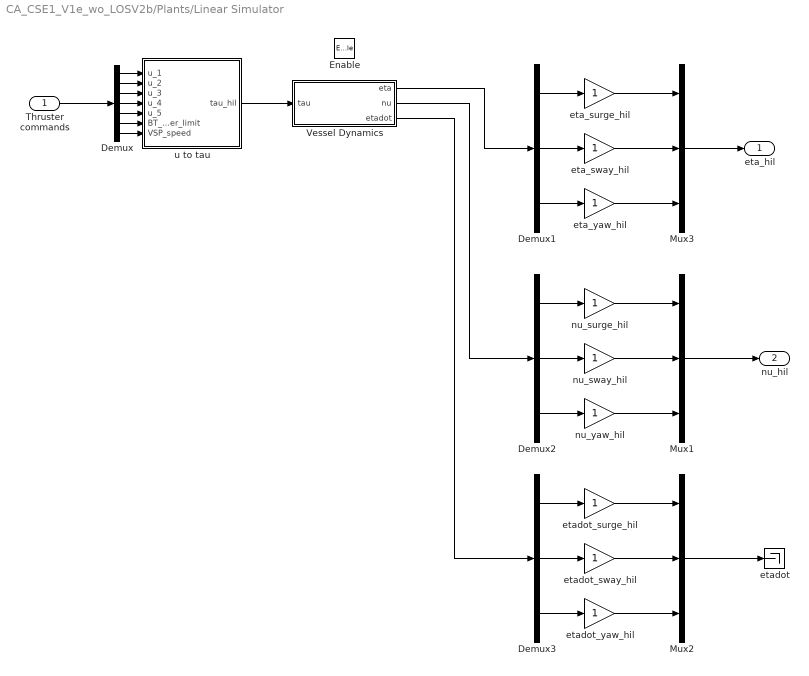
== system CA_CSE1_V1e_wo_LOSV2b/Plants/Linear Simulator ==
  Thruster commands : Inport
  Enable : EnablePort  StatesWhenEnabling=reset
  Demux : Demux  Outputs=7
  Demux1 : Demux  Outputs=3
  Demux2 : Demux  Outputs=3
  Demux3 : Demux  Outputs=3
  Mux1 : Mux  Inputs=3
  Mux2 : Mux  Inputs=3
  Mux3 : Mux  Inputs=3
  Vessel Dynamics : Subsystem
  eta_surge_hil : Gain  ParameterDataType=fixdt(1, 16)  ParameterScaling=2^0  OutDataType=fixdt(1, 16)  OutScaling=2^0
  eta_sway_hil : Gain  ParameterDataType=fixdt(1, 16)  ParameterScaling=2^0  OutDataType=fixdt(1, 16)  OutScaling=2^0
  eta_yaw_hil : Gain  ParameterDataType=fixdt(1, 16)  ParameterScaling=2^0  OutDataType=fixdt(1, 16)  OutScaling=2^0
  etadot : Terminator
  etadot_surge_hil : Gain  ParameterDataType=fixdt(1, 16)  ParameterScaling=2^0  OutDataType=fixdt(1, 16)  OutScaling=2^0
  etadot_sway_hil : Gain  ParameterDataType=fixdt(1, 16)  ParameterScaling=2^0  OutDataType=fixdt(1, 16)  OutScaling=2^0
  etadot_yaw_hil : Gain  ParameterDataType=fixdt(1, 16)  ParameterScaling=2^0  OutDataType=fixdt(1, 16)  OutScaling=2^0
  nu_surge_hil : Gain  ParameterDataType=fixdt(1, 16)  ParameterScaling=2^0  OutDataType=fixdt(1, 16)  OutScaling=2^0
  nu_sway_hil : Gain  ParameterDataType=fixdt(1, 16)  ParameterScaling=2^0  OutDataType=fixdt(1, 16)  OutScaling=2^0
  nu_yaw_hil : Gain  ParameterDataType=fixdt(1, 16)  ParameterScaling=2^0  OutDataType=fixdt(1, 16)  OutScaling=2^0
  u to tau : Subsystem
  eta_hil : Outport
  nu_hil : Outport  Port=2
  wires:
  Thruster commands/1 -> Demux/1
  u to tau/1(tau_hil) -> Vessel Dynamics/1(tau)
  Demux/1 -> u to tau/1(u_1)
  Demux/2 -> u to tau/2(u_2)
  Demux/3 -> u to tau/3(u_3)
  Demux/4 -> u to tau/4(u_4)
  Demux/5 -> u to tau/5(u_5)
  Demux/6 -> u to tau/6(BT_power_limit)
  Demux/7 -> u to tau/7(VSP_speed)
  nu_yaw_hil/1 -> Mux1/3
  nu_sway_hil/1 -> Mux1/2
  nu_surge_hil/1 -> Mux1/1
  Demux2/3 -> nu_yaw_hil/1
  Demux2/2 -> nu_sway_hil/1
  Demux2/1 -> nu_surge_hil/1
  eta_sway_hil/1 -> Mux3/2
  eta_yaw_hil/1 -> Mux3/3
  eta_surge_hil/1 -> Mux3/1
  Demux1/3 -> eta_yaw_hil/1
  Demux1/2 -> eta_sway_hil/1
  Demux1/1 -> eta_surge_hil/1
  Vessel Dynamics/1(eta) -> Demux1/1
  Vessel Dynamics/2(nu) -> Demux2/1
  Mux1/1 -> nu_hil/1
  Mux3/1 -> eta_hil/1
  etadot_sway_hil/1 -> Mux2/2
  etadot_yaw_hil/1 -> Mux2/3
  etadot_surge_hil/1 -> Mux2/1
  Demux3/3 -> etadot_yaw_hil/1
  Demux3/2 -> etadot_sway_hil/1
  Demux3/1 -> etadot_surge_hil/1
  Vessel Dynamics/3(etadot) -> Demux3/1
  Mux2/1 -> etadot/1

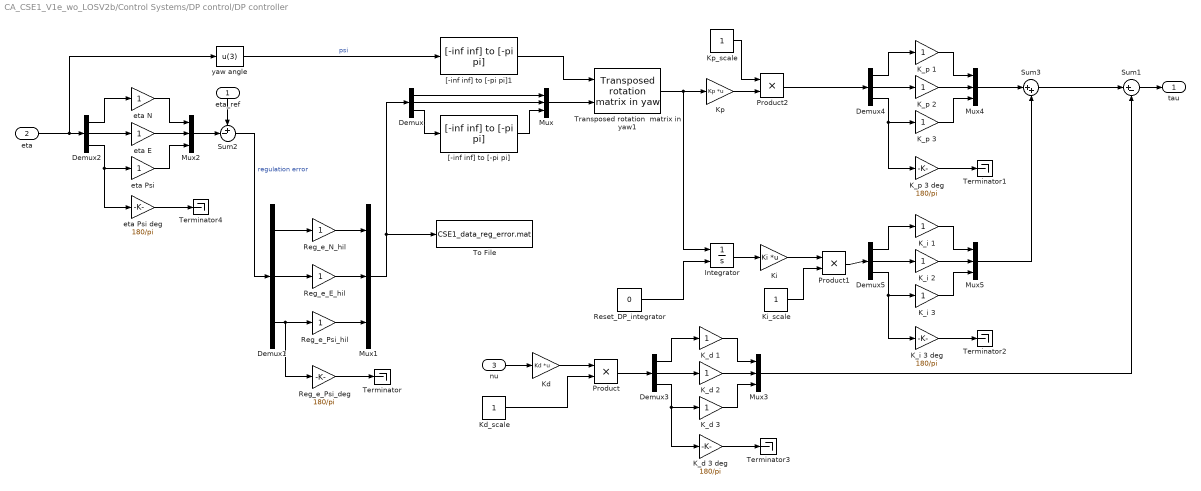
== system CA_CSE1_V1e_wo_LOSV2b/Control Systems/DP control/DP controller ==
  eta_ref : Inport
  eta : Inport  Port=2
  nu : Inport  Port=3
  Demux{,1..5} (6 alike) : Demux  Outputs=3
  Integrator : Integrator  ExternalReset=level
  K_d 1 : Gain  ParameterDataType=fixdt(1, 16)  ParameterScaling=2^0  OutDataType=fixdt(1, 16)  OutScaling=2^0
  K_d 2 : Gain  ParameterDataType=fixdt(1, 16)  ParameterScaling=2^0  OutDataType=fixdt(1, 16)  OutScaling=2^0
  K_d 3 : Gain  ParameterDataType=fixdt(1, 16)  ParameterScaling=2^0  OutDataType=fixdt(1, 16)  OutScaling=2^0
  K_d 3 deg : Gain  Gain=180/pi  ParameterDataType=fixdt(1, 16)  ParameterScaling=2^0  OutDataType=fixdt(1, 16)  OutScaling=2^0
  K_i 1 : Gain  ParameterDataType=fixdt(1, 16)  ParameterScaling=2^0  OutDataType=fixdt(1, 16)  OutScaling=2^0
  K_i 2 : Gain  ParameterDataType=fixdt(1, 16)  ParameterScaling=2^0  OutDataType=fixdt(1, 16)  OutScaling=2^0
  K_i 3 : Gain  ParameterDataType=fixdt(1, 16)  ParameterScaling=2^0  OutDataType=fixdt(1, 16)  OutScaling=2^0
  K_i 3 deg : Gain  Gain=180/pi  ParameterDataType=fixdt(1, 16)  ParameterScaling=2^0  OutDataType=fixdt(1, 16)  OutScaling=2^0
  K_p 1 : Gain  ParameterDataType=fixdt(1, 16)  ParameterScaling=2^0  OutDataType=fixdt(1, 16)  OutScaling=2^0
  K_p 2 : Gain  ParameterDataType=fixdt(1, 16)  ParameterScaling=2^0  OutDataType=fixdt(1, 16)  OutScaling=2^0
  K_p 3 : Gain  ParameterDataType=fixdt(1, 16)  ParameterScaling=2^0  OutDataType=fixdt(1, 16)  OutScaling=2^0
  K_p 3 deg : Gain  Gain=180/pi  ParameterDataType=fixdt(1, 16)  ParameterScaling=2^0  OutDataType=fixdt(1, 16)  OutScaling=2^0
  Kd : Gain  Gain=Kd  Multiplication=Matrix(K*u)  SaturateOnIntegerOverflow=on  OutDataTypeStr=Inherit: Same as input  ParamDataTypeStr=Inherit: Same as input
  Kd_scale : Constant
  Ki : Gain  Gain=Ki  Multiplication=Matrix(K*u)  SaturateOnIntegerOverflow=on  OutDataTypeStr=Inherit: Same as input  ParamDataTypeStr=Inherit: Same as input
  Ki_scale : Constant
  Kp : Gain  Gain=Kp  Multiplication=Matrix(K*u)  SaturateOnIntegerOverflow=on  OutDataTypeStr=Inherit: Same as input  ParamDataTypeStr=Inherit: Same as input
  Kp_scale : Constant
  Mux{,1..5} (6 alike) : Mux  Inputs=3
  Product : Product  RndMeth=Zero
  Product1 : Product  RndMeth=Zero
  Product2 : Product  RndMeth=Zero
  Reg_e_E_hil : Gain
  Reg_e_N_hil : Gain
  Reg_e_Psi_deg : Gain  Gain=180/pi  ParameterDataType=fixdt(1, 16)  ParameterScaling=2^0  OutDataType=fixdt(1, 16)  OutScaling=2^0
  Reg_e_Psi_hil : Gain
  Reset_DP_integrator : Constant  Value=0
  Sum1 : Sum  Inputs=|+-  SaturateOnIntegerOverflow=on  InputSameDT=on  OutDataTypeStr=Inherit: Same as first input
  Sum2 : Sum  Inputs=+-|  SaturateOnIntegerOverflow=on  InputSameDT=on  OutDataTypeStr=Inherit: Same as first input
  Sum3 : Sum  Inputs=|++  SaturateOnIntegerOverflow=on  InputSameDT=on  OutDataTypeStr=Inherit: Same as first input
  Terminator{,1..4} (5 alike) : Terminator
  To File : ToFile  Filename=CSE1_data_reg_error.mat  MatrixName=cse1_data_reg_error
  Transposed rotation  matrix in yaw1 : marine_gnc/Models/ Kinematics/Transposed rotation  matrix in yaw  SystemSampleTime=-1
  "[-inf inf] to [-pi pi]" : marine_gnc/Utilities/Math Operations/[-inf inf] to [-pi pi]  SystemSampleTime=-1
  "[-inf inf] to [-pi pi]1" : marine_gnc/Utilities/Math Operations/[-inf inf] to [-pi pi]  SystemSampleTime=-1
  eta E : Gain  ParameterDataType=fixdt(1, 16)  ParameterScaling=2^0  OutDataType=fixdt(1, 16)  OutScaling=2^0
  eta N : Gain  ParameterDataType=fixdt(1, 16)  ParameterScaling=2^0  OutDataType=fixdt(1, 16)  OutScaling=2^0
  eta Psi : Gain  ParameterDataType=fixdt(1, 16)  ParameterScaling=2^0  OutDataType=fixdt(1, 16)  OutScaling=2^0
  eta Psi deg : Gain  Gain=180/pi  ParameterDataType=fixdt(1, 16)  ParameterScaling=2^0  OutDataType=fixdt(1, 16)  OutScaling=2^0
  yaw angle : Fcn  Expr=u(3)
  tau : Outport  InitialOutput=0
  wires:
  Mux/1 -> Transposed rotation  matrix in yaw1/2
  Demux/1 -> Mux/1
  Demux/2 -> Mux/2
  eta_ref/1 -> Sum2/1
  Sum1/1 -> tau/1
  eta/1 -> yaw angle/1, Demux2/1
  Integrator/1 -> Ki/1
  Sum3/1 -> Sum1/1
  Transposed rotation  matrix in yaw1/1 -> Kp/1, Integrator/1
  Demux1/1 -> Reg_e_N_hil/1
  Reg_e_N_hil/1 -> Mux1/1
  Sum2/1 -> Demux1/1  "regulation error"
  Demux1/2 -> Reg_e_E_hil/1
  Reg_e_E_hil/1 -> Mux1/2
  Demux1/3 -> Reg_e_Psi_hil/1, Reg_e_Psi_deg/1
  Reg_e_Psi_hil/1 -> Mux1/3
  Mux1/1 -> Demux/1, To File/1
  nu/1 -> Kd/1
  Kd/1 -> Product/1
  Kd_scale/1 -> Product/2
  Ki/1 -> Product1/1
  Ki_scale/1 -> Product1/2
  Kp/1 -> Product2/2
  Kp_scale/1 -> Product2/1
  Reset_DP_integrator/1 -> Integrator/2
  yaw angle/1 -> "[-inf inf] to [-pi pi]1"/1  "psi"
  "[-inf inf] to [-pi pi]1"/1 -> Transposed rotation  matrix in yaw1/1
  Demux/3 -> "[-inf inf] to [-pi pi]"/1
  "[-inf inf] to [-pi pi]"/1 -> Mux/3
  eta N/1 -> Mux2/1
  eta E/1 -> Mux2/2
  eta Psi/1 -> Mux2/3
  Demux2/1 -> eta N/1
  Demux2/2 -> eta E/1
  Demux2/3 -> eta Psi/1, eta Psi deg/1
  Mux2/1 -> Sum2/2
  K_d 1/1 -> Mux3/1
  K_d 2/1 -> Mux3/2
  K_d 3/1 -> Mux3/3
  Demux3/1 -> K_d 1/1
  Demux3/2 -> K_d 2/1
  Demux3/3 -> K_d 3/1, K_d 3 deg/1
  Product/1 -> Demux3/1
  Mux3/1 -> Sum1/2
  K_p 1/1 -> Mux4/1
  K_p 2/1 -> Mux4/2
  K_p 3/1 -> Mux4/3
  Demux4/1 -> K_p 1/1
  Demux4/2 -> K_p 2/1
  Demux4/3 -> K_p 3/1, K_p 3 deg/1
  Product2/1 -> Demux4/1
  Mux4/1 -> Sum3/1
  K_i 1/1 -> Mux5/1
  K_i 2/1 -> Mux5/2
  K_i 3/1 -> Mux5/3
  Demux5/1 -> K_i 1/1
  Demux5/2 -> K_i 2/1
  Demux5/3 -> K_i 3/1, K_i 3 deg/1
  Product1/1 -> Demux5/1
  Mux5/1 -> Sum3/2
  K_p 3 deg/1 -> Terminator1/1
  K_i 3 deg/1 -> Terminator2/1
  K_d 3 deg/1 -> Terminator3/1
  Reg_e_Psi_deg/1 -> Terminator/1
  eta Psi deg/1 -> Terminator4/1

== system CA_CSE1_V1e_wo_LOSV2b/Control Systems/DP control/K_e ==
  Constant : Constant  Value=0  OutDataType=fixdt(1, 16)  OutScaling=2^0
  Gain K_e1_DP : Gain  ParameterDataType=fixdt(1, 16)  ParameterScaling=2^0  OutDataType=fixdt(1, 16)  OutScaling=2^0
  Gain K_e2_DP : Gain  ParameterDataType=fixdt(1, 16)  ParameterScaling=2^0  OutDataType=fixdt(1, 16)  OutScaling=2^0
  Gain K_e3_DP : Gain  ParameterDataType=fixdt(1, 16)  ParameterScaling=2^0  OutDataType=fixdt(1, 16)  OutScaling=2^0
  Gain K_e4_DP : Gain  ParameterDataType=fixdt(1, 16)  ParameterScaling=2^0  OutDataType=fixdt(1, 16)  OutScaling=2^0
  Gain K_e5_DP : Gain  ParameterDataType=fixdt(1, 16)  ParameterScaling=2^0  OutDataType=fixdt(1, 16)  OutScaling=2^0
  K_e1_DP : Constant  OutDataType=fixdt(1, 16)  OutScaling=2^0
  K_e2_DP : Constant  OutDataType=fixdt(1, 16)  OutScaling=2^0
  K_e3_DP : Constant  OutDataType=fixdt(1, 16)  OutScaling=2^0
  K_e4_DP : Constant  OutDataType=fixdt(1, 16)  OutScaling=2^0
  K_e5_DP : Constant  OutDataType=fixdt(1, 16)  OutScaling=2^0
  Mux12 : Mux  Inputs=25
  Thruster Gain matrix : Reshape  OutputDimensionality=Customize  OutputDimensions=[5,5]
  K_e : Outport  OutDataType=fixdt(1, 16)  OutScaling=2^0
  wires:
  Mux12/1 -> Thruster Gain matrix/1
  K_e1_DP/1 -> Gain K_e1_DP/1
  Thruster Gain matrix/1 -> K_e/1
  Constant/1 -> Mux12/4, Mux12/2, Mux12/3, Mux12/5, Mux12/6, Mux12/8, Mux12/9, Mux12/10, Mux12/11, Mux12/12, Mux12/14, Mux12/15, Mux12/16, Mux12/17, Mux12/18, Mux12/20, Mux12/21, Mux12/22, Mux12/23, Mux12/24
  K_e2_DP/1 -> Gain K_e2_DP/1
  K_e3_DP/1 -> Gain K_e3_DP/1
  K_e4_DP/1 -> Gain K_e4_DP/1
  K_e5_DP/1 -> Gain K_e5_DP/1
  Gain K_e1_DP/1 -> Mux12/1
  Gain K_e2_DP/1 -> Mux12/7
  Gain K_e3_DP/1 -> Mux12/13
  Gain K_e4_DP/1 -> Mux12/19
  Gain K_e5_DP/1 -> Mux12/25

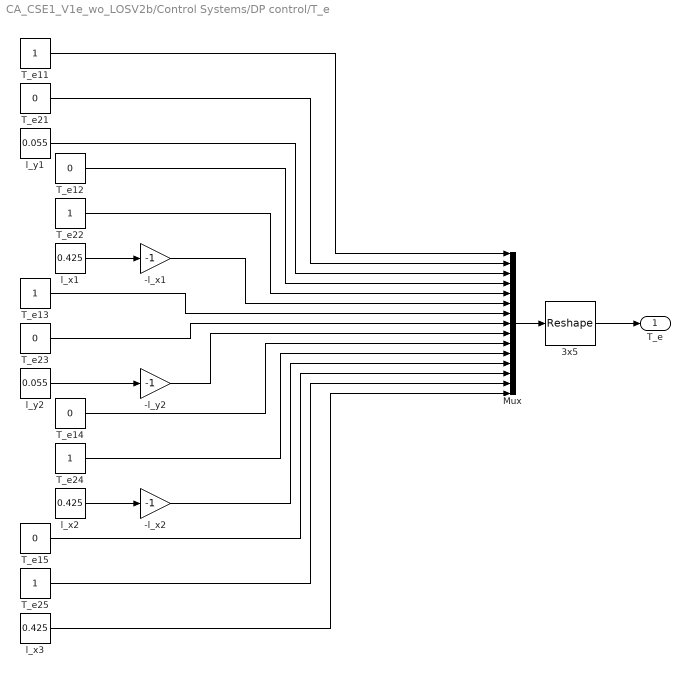
== system CA_CSE1_V1e_wo_LOSV2b/Control Systems/DP control/T_e ==
  -l_x1 : Gain  Gain=-1
  -l_x2 : Gain  Gain=-1
  -l_y2 : Gain  Gain=-1
  3x5 : Reshape  OutputDimensionality=Customize  OutputDimensions=[3,5]
  Mux : Mux  Inputs=15
  T_e{11,13,22,24..25} (5 alike) : Constant
  T_e{12,14..15,21,23} (5 alike) : Constant  Value=0
  l_x1 : Constant  Value=0.425
  l_x2 : Constant  Value=0.425
  l_x3 : Constant  Value=0.425
  l_y1 : Constant  Value=0.055
  l_y2 : Constant  Value=0.055
  T_e : Outport
  wires:
  Mux/1 -> 3x5/1
  3x5/1 -> T_e/1
  T_e11/1 -> Mux/1
  T_e21/1 -> Mux/2
  l_y1/1 -> Mux/3
  T_e12/1 -> Mux/4
  T_e22/1 -> Mux/5
  l_x1/1 -> -l_x1/1
  T_e13/1 -> Mux/7
  T_e23/1 -> Mux/8
  l_y2/1 -> -l_y2/1
  T_e14/1 -> Mux/10
  T_e24/1 -> Mux/11
  l_x2/1 -> -l_x2/1
  T_e15/1 -> Mux/13
  T_e25/1 -> Mux/14
  l_x3/1 -> Mux/15
  -l_x1/1 -> Mux/6
  -l_y2/1 -> Mux/9
  -l_x2/1 -> Mux/12

== system CA_CSE1_V1e_wo_LOSV2b/Control Systems/Joystick Control/K_e ==
  Constant : Constant  Value=0  OutDataType=fixdt(1, 16)  OutScaling=2^0
  Gain K_e1_joystick : Gain  ParameterDataType=fixdt(1, 16)  ParameterScaling=2^0  OutDataType=fixdt(1, 16)  OutScaling=2^0
  Gain K_e2_joystick : Gain  ParameterDataType=fixdt(1, 16)  ParameterScaling=2^0  OutDataType=fixdt(1, 16)  OutScaling=2^0
  Gain K_e3_joystick : Gain  ParameterDataType=fixdt(1, 16)  ParameterScaling=2^0  OutDataType=fixdt(1, 16)  OutScaling=2^0
  Gain K_e4_joystick : Gain  ParameterDataType=fixdt(1, 16)  ParameterScaling=2^0  OutDataType=fixdt(1, 16)  OutScaling=2^0
  Gain K_e5_joystick : Gain  ParameterDataType=fixdt(1, 16)  ParameterScaling=2^0  OutDataType=fixdt(1, 16)  OutScaling=2^0
  K_e1_joystick : Constant  OutDataType=fixdt(1, 16)  OutScaling=2^0
  K_e2_joystick : Constant  OutDataType=fixdt(1, 16)  OutScaling=2^0
  K_e3_joystick : Constant  OutDataType=fixdt(1, 16)  OutScaling=2^0
  K_e4_joystick : Constant  OutDataType=fixdt(1, 16)  OutScaling=2^0
  K_e5_joystick : Constant  OutDataType=fixdt(1, 16)  OutScaling=2^0
  Mux12 : Mux  Inputs=25
  Thruster Gain matrix : Reshape  OutputDimensionality=Customize  OutputDimensions=[5,5]
  K_e : Outport  OutDataType=fixdt(1, 16)  OutScaling=2^0
  wires:
  Mux12/1 -> Thruster Gain matrix/1
  K_e1_joystick/1 -> Gain K_e1_joystick/1
  Thruster Gain matrix/1 -> K_e/1
  Constant/1 -> Mux12/4, Mux12/2, Mux12/3, Mux12/5, Mux12/6, Mux12/8, Mux12/9, Mux12/10, Mux12/11, Mux12/12, Mux12/14, Mux12/15, Mux12/16, Mux12/17, Mux12/18, Mux12/20, Mux12/21, Mux12/22, Mux12/23, Mux12/24
  K_e2_joystick/1 -> Gain K_e2_joystick/1
  K_e3_joystick/1 -> Gain K_e3_joystick/1
  K_e4_joystick/1 -> Gain K_e4_joystick/1
  K_e5_joystick/1 -> Gain K_e5_joystick/1
  Gain K_e1_joystick/1 -> Mux12/1
  Gain K_e2_joystick/1 -> Mux12/7
  Gain K_e3_joystick/1 -> Mux12/13
  Gain K_e4_joystick/1 -> Mux12/19
  Gain K_e5_joystick/1 -> Mux12/25

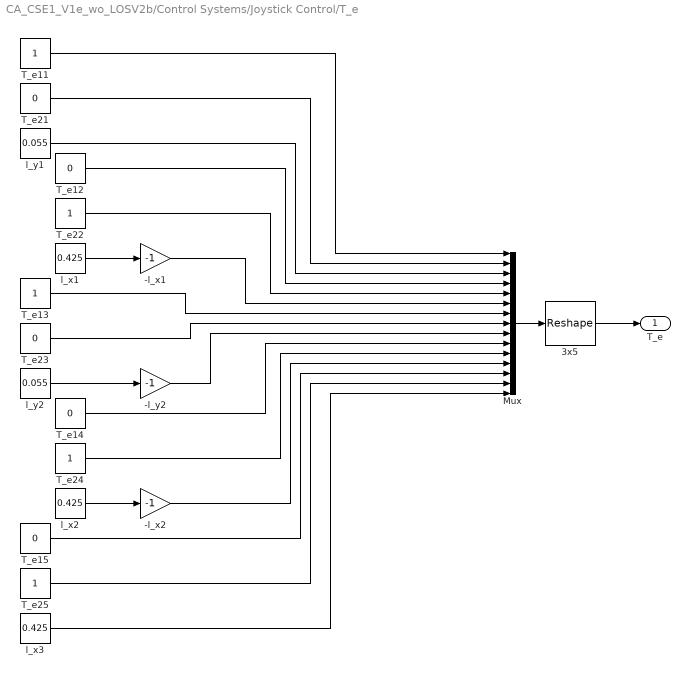
== system CA_CSE1_V1e_wo_LOSV2b/Control Systems/Joystick Control/T_e ==
  -l_x1 : Gain  Gain=-1
  -l_x2 : Gain  Gain=-1
  -l_y2 : Gain  Gain=-1
  3x5 : Reshape  OutputDimensionality=Customize  OutputDimensions=[3,5]
  Mux : Mux  Inputs=15
  T_e{11,13,22,24..25} (5 alike) : Constant
  T_e{12,14..15,21,23} (5 alike) : Constant  Value=0
  l_x1 : Constant  Value=0.425
  l_x2 : Constant  Value=0.425
  l_x3 : Constant  Value=0.425
  l_y1 : Constant  Value=0.055
  l_y2 : Constant  Value=0.055
  T_e : Outport
  wires:
  Mux/1 -> 3x5/1
  3x5/1 -> T_e/1
  T_e11/1 -> Mux/1
  T_e21/1 -> Mux/2
  l_y1/1 -> Mux/3
  T_e12/1 -> Mux/4
  T_e22/1 -> Mux/5
  l_x1/1 -> -l_x1/1
  T_e13/1 -> Mux/7
  T_e23/1 -> Mux/8
  l_y2/1 -> -l_y2/1
  T_e14/1 -> Mux/10
  T_e24/1 -> Mux/11
  l_x2/1 -> -l_x2/1
  T_e15/1 -> Mux/13
  T_e25/1 -> Mux/14
  l_x3/1 -> Mux/15
  -l_x1/1 -> Mux/6
  -l_y2/1 -> Mux/9
  -l_x2/1 -> Mux/12

== system CA_CSE1_V1e_wo_LOSV2b/HMI/PS3 input/PS3 signals ==
  note: PS3 signals
  note: R2 Button
  note: L2 Button
  note: Normalized
  note: Normalized
  note: Normalized
  note: Normalized
  note: Up/Down position of Right Joystick
  note: Left/Right position of Right Joystick
  note: Up/Down position of Left Joystick
  note: Left/Right position of Left Joystick
  JS_L_X : Constant  Value=0
  JS_L_Y : Constant  Value=0
  JS_R_X : Constant  Value=0
  JS_R_Y : Constant  Value=0
  L2 : Constant  Value=0
  Mux : Mux  Inputs=6
  R2 : Constant  Value=0
  Scaling_JS_L_X : Gain  Gain=1/32767
  Scaling_JS_L_Y : Gain  Gain=1/32767
  Scaling_JS_R_X : Gain  Gain=1/32767
  Scaling_JS_R_Y : Gain  Gain=1/32767
  PS3 signals : Outport
  wires:
  Mux/1 -> PS3 signals/1
  JS_L_X/1 -> Scaling_JS_L_X/1  "[-32767,32767]"
  Scaling_JS_L_X/1 -> Mux/1  "[-1,1]"
  JS_L_Y/1 -> Scaling_JS_L_Y/1  "[-32767,32767]"
  Scaling_JS_L_Y/1 -> Mux/2  "[-1,1]"
  JS_R_X/1 -> Scaling_JS_R_X/1  "[-32767,32767]"
  Scaling_JS_R_X/1 -> Mux/3  "[-1,1]"
  Scaling_JS_R_Y/1 -> Mux/4  "[-1,1]"
  JS_R_Y/1 -> Scaling_JS_R_Y/1  "[-32767,32767]"
  L2/1 -> Mux/5  "[-1,0]"
  R2/1 -> Mux/6  "[0,1]"

== system CA_CSE1_V1e_wo_LOSV2b/Plants/CSE1/Bow Thruster ==
  Bow Thruster Direction u_5 : Inport
  Bow Thruster Power : Inport  Port=2
  Add : Sum  Inputs=+++
  BT_D_Gain1 : Gain  Gain=0.02
  BT_D_Gain2 : Gain  Gain=0.02
  BT_L_Gain1 : Gain  Gain=0.02
  BT_L_Gain2 : Gain  Gain=-0.02
  BT_Power_Offset1 : Constant  Value=0.05
  BT_Power_Offset2 : Constant  Value=0.05
  BT_Power_Offset3 : Constant  Value=0.05
  Constant : Constant  Value=0  OutDataType=fixdt(1, 16)  OutScaling=2^0
  Constant1 : Constant  Value=0  OutDataType=fixdt(1, 16)  OutScaling=2^0
  Neg : Gain  Gain=-1  ParameterDataType=fixdt(1, 16)  ParameterScaling=2^0  OutDataType=fixdt(1, 16)  OutScaling=2^0
  SIT Out5 BT : S-Function  Priority=1  FunctionName=NI_SIT_IO  Parameters=width dtype portnum stime stype btype  EnableBusSupport=off  mask(SIT Outport){portnum=1, width=-1, stime=-1, dtype=auto, stype=auto, btype=0}
      mask prompts: portnum "Port number:"; width "Port dimensions (-1 for dynamically sized):"; stime "Sample time (-1 for inherited):"; dtype "Data type:"; stype "Signal type:"; btype "Block type:"
      mask help: Use this outport on any level of nested subsystems to allow the LabVIEW Simulation Interface Toolkit to map hardware to it.
      mask init:
      | NI_SIT_IO_init;
      settings: CopyFcn=NI_SIT_IO_callbacks(1);  DeleteFcn=NI_SIT_IO_callbacks(2);
      mask StyleString: edit,edit,edit,popup(auto|double|single|int8|uint8|int16|uint16|int32|uint32|boolean),popup(auto|real|complex),edit
      mask CallbackString: NI_SIT_IO_callbacks(3);|||NI_SIT_IO_callbacks(4);||
      mask TabNameString: Parameters,Parameters,Parameters,Parameters,Parameters,Parameters
      mask Display:
      | patch([-x x], [-y y], [.90980 .81960 .32156]);
      | plot([0 -x x 0], [rad -y y rad]);
      | fprintf('SIT%d', portnum);
  Saturation Dynamic : simulink/Discontinuities/Saturation Dynamic  SystemSampleTime=-1  OutMin=[]  OutMax=[]  OutDataTypeStr=Inherit: Same as second input  OutDataType=fixdt(1, 16)  OutScaling=2^-10  DoSatur=off
  Saturation Dynamic1 : simulink/Discontinuities/Saturation Dynamic  SystemSampleTime=-1  OutMin=[]  OutMax=[]  OutDataTypeStr=Inherit: Same as second input  OutDataType=fixdt(1, 16)  OutScaling=2^-10  DoSatur=off
  Saturation Dynamic2 : simulink/Discontinuities/Saturation Dynamic  SystemSampleTime=-1  OutMin=[]  OutMax=[]  OutDataTypeStr=Inherit: Same as second input  OutDataType=fixdt(1, 16)  OutScaling=2^-10  DoSatur=off
  Sum1 : Sum  Inputs=|++
  Sum2 : Sum  Inputs=|++
  Terminator : Terminator
  Terminator1 : Terminator
  wires:
  Bow Thruster Direction u_5/1 -> BT_D_Gain1/1, Saturation Dynamic1/2, BT_D_Gain2/1, Saturation Dynamic2/2
  BT_D_Gain1/1 -> Add/1
  BT_D_Gain2/1 -> Add/3
  BT_Power_Offset1/1 -> Add/2
  Add/1 -> Saturation Dynamic/2
  Bow Thruster Power/1 -> BT_L_Gain2/1, Saturation Dynamic2/1, BT_L_Gain1/1, Neg/1
  Sum1/1 -> Saturation Dynamic/1
  BT_L_Gain1/1 -> Sum1/1
  BT_L_Gain2/1 -> Sum2/1
  Sum2/1 -> Saturation Dynamic/3
  BT_Power_Offset2/1 -> Sum1/2
  BT_Power_Offset3/1 -> Sum2/2
  Saturation Dynamic/1 -> SIT Out5 BT/1
  Saturation Dynamic2/1 -> Terminator1/1
  Saturation Dynamic1/1 -> Terminator/1
  Constant/1 -> Saturation Dynamic1/1
  Constant1/1 -> Saturation Dynamic2/3
  Neg/1 -> Saturation Dynamic1/3
